simulink model "QPSK_UDP_Print"  (R2017b)
settings: Solver=VariableStepAuto  StartTime=0.0  StopTime=inf  RelTol=1e-3
libraries: dspnetwork x1
settings Model: Creator=The MathWorks, Inc.  LastModifiedBy=ppradhan
settings CodeAppCC: StateflowObjectComments=on

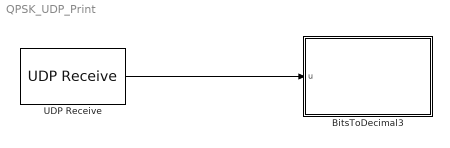
== system QPSK_UDP_Print ==
  BitsToDecimal3 : MATLAB Function  TreatAsAtomicUnit=on
  UDP Receive : dspnetwork/UDP Receive  localURL='0.0.0.0'  localPort=25000  remoteURL='0.0.0.0'  remotePort=-1  recvBufferSize=24*1000  dims=24  signalDatatype=int8  isVarSize=on  showBlockingTime=off  blockingTime=0  sampletime=1/100e3  blockPlatform=[]
      settings: SourceProductName=DSP System Toolbox  SourceProductBaseCode=DS
  wires:
  UDP Receive/1 -> BitsToDecimal3/1(u)

== matlab function QPSK_UDP_Print/BitsToDecimal3 ==
  data: u input
function UDPHostPrintf(u)
% Display ASCII message to command window

fprintf('%s\n',char(u));
